simulink model "ModeloMonza"  (R2020b)
settings: Solver=FixedStepAuto  StartTime=0.0  StopTime=7  FixedStep=0.001  RelTol=1e-3
undefined symbols (not defined in the file or in its folder): magnitude
libraries: simulink x2, simulink_extras x1
settings Model: PauseTimes=2.78  Creator=alvar  LastModifiedBy=alvar
settings SolverCC: AlgebraicLoopSolver=LineSearch

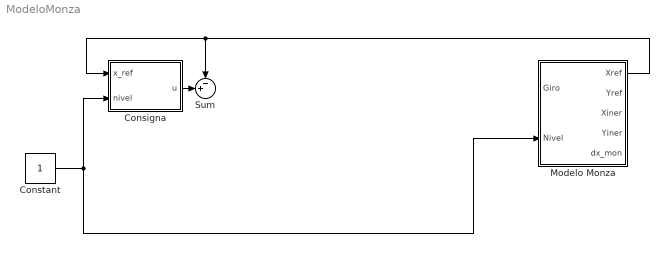
== system ModeloMonza ==
  Consigna : MATLAB Function  TreatAsAtomicUnit=on
  Constant : Constant
  Modelo Monza : Subsystem
  Sum : Sum  Inputs=-+|
  wires:
  Constant/1 -> Modelo Monza/2(Nivel), Consigna/2(nivel)
  Modelo Monza/1(Xref) -> Consigna/1(x_ref), Sum/1
  Consigna/1(u) -> Sum/2

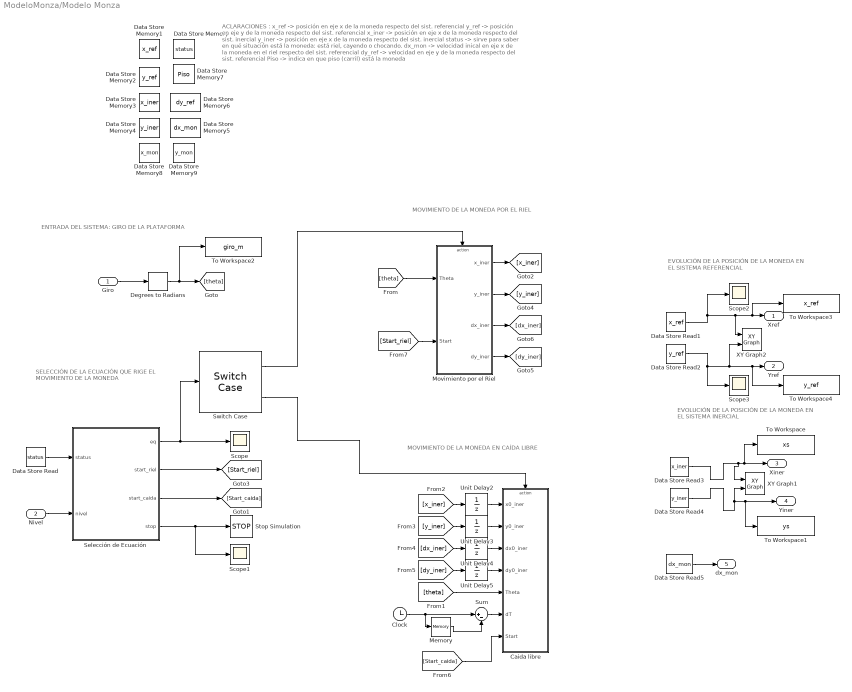
== system ModeloMonza/Modelo Monza ==
  note: ENTRADA DEL SISTEMA: GIRO DE LA PLATAFORMA
  note: SELECCIÓN DE LA ECUACIÓN QUE RIGE EL MOVIMIENTO DE LA MONEDA
  note: MOVIMIENTO DE LA MONEDA EN CAÍDA LIBRE
  note: MOVIMIENTO DE LA MONEDA POR EL RIEL
  note: EVOLUCIÓN DE LA POSICIÓN DE LA MONEDA EN EL SISTEMA REFERENCIAL
  note: ACLARACIONES :
      |
      | x_ref -> posición en eje x de la moneda respecto del sist. referencial
      | y_ref -> posición en eje y de la moneda respecto del sist. referencial
      |
      | x_iner -> posición en eje x de la moneda respecto del sist. inercial
      | y_iner -> posición en eje x de la moneda respecto del sist. inercial
      |
      | status -> sirve para saber en qué situación está la moneda: está riel, cayendo o chocando.
      |
      | dx_mon -> velocidad inical en eje x de la moneda en el riel respecto del sist. referencial
      |
      | dy_ref -> velocidad en eje y de la moneda respecto del sist. referencial
      |
      | Piso -> indica en que piso (carril) está la moneda
  note: EVOLUCIÓN DE LA POSICIÓN DE LA MONEDA EN EL SISTEMA INERCIAL
  Giro : Inport
  Nivel : Inport  Port=2
  Caida libre : Subsystem  TreatAsAtomicUnit=on
  Clock : Clock
  Data Store Memory : DataStoreMemory  DataStoreName=status  ReadBeforeWriteMsg=warning  WriteAfterWriteMsg=warning  WriteAfterReadMsg=warning  ShowAdditionalParam=off  OutDataTypeStr=double
  Data Store Memory1 : DataStoreMemory  DataStoreName=x_ref  ReadBeforeWriteMsg=warning  WriteAfterWriteMsg=warning  WriteAfterReadMsg=warning  InitialValue=-0.11  ShowAdditionalParam=off  OutDataTypeStr=double
  Data Store Memory2 : DataStoreMemory  DataStoreName=y_ref  ReadBeforeWriteMsg=warning  WriteAfterWriteMsg=warning  WriteAfterReadMsg=warning  InitialValue=0.107766  ShowAdditionalParam=off  OutDataTypeStr=double
  Data Store Memory3 : DataStoreMemory  DataStoreName=x_iner  ReadBeforeWriteMsg=warning  WriteAfterWriteMsg=warning  WriteAfterReadMsg=warning  InitialValue=-0.11  ShowAdditionalParam=off  OutDataTypeStr=double
  Data Store Memory4 : DataStoreMemory  DataStoreName=y_iner  ReadBeforeWriteMsg=warning  WriteAfterWriteMsg=warning  WriteAfterReadMsg=warning  InitialValue=0.107766  ShowAdditionalParam=off  OutDataTypeStr=double
  Data Store Memory5 : DataStoreMemory  DataStoreName=dx_mon  ReadBeforeWriteMsg=warning  WriteAfterWriteMsg=warning  WriteAfterReadMsg=warning  ShowAdditionalParam=off  OutDataTypeStr=double
  Data Store Memory6 : DataStoreMemory  DataStoreName=dy_ref  ReadBeforeWriteMsg=warning  WriteAfterWriteMsg=warning  WriteAfterReadMsg=warning  ShowAdditionalParam=off  OutDataTypeStr=double
  Data Store Memory7 : DataStoreMemory  DataStoreName=Piso  ReadBeforeWriteMsg=warning  WriteAfterWriteMsg=warning  WriteAfterReadMsg=warning  InitialValue=1  ShowAdditionalParam=off  OutDataTypeStr=double
  Data Store Memory8 : DataStoreMemory  DataStoreName=x_mon  ReadBeforeWriteMsg=warning  WriteAfterWriteMsg=warning  WriteAfterReadMsg=warning  InitialValue=-0.11  ShowAdditionalParam=off  OutDataTypeStr=double
  Data Store Memory9 : DataStoreMemory  DataStoreName=y_mon  ReadBeforeWriteMsg=warning  WriteAfterWriteMsg=warning  WriteAfterReadMsg=warning  InitialValue=0.107766  ShowAdditionalParam=off  OutDataTypeStr=double
  Data Store Read : DataStoreRead  DataStoreName=status
  Data Store Read1 : DataStoreRead  DataStoreName=x_ref
  Data Store Read2 : DataStoreRead  DataStoreName=y_ref
  Data Store Read3 : DataStoreRead  DataStoreName=x_iner
  Data Store Read4 : DataStoreRead  DataStoreName=y_iner
  Data Store Read5 : DataStoreRead  DataStoreName=dx_mon
  Degrees to Radians : simulink_extras/Transformations/Degrees to Radians
  Memory : Memory
  Movimiento por el Riel : Subsystem  TreatAsAtomicUnit=on
  Scope{,1..3} (4 alike) : Scope
  Selección de Ecuación : MATLAB Function  TreatAsAtomicUnit=on
  Stop Simulation : Stop
  Sum : Sum  Inputs=|+-
  Switch Case : SwitchCase  CaseConditions={1,2}  ShowDefaultCase=off
  To Workspace : ToWorkspace  VariableName=xs  SampleTime=0.01
  To Workspace1 : ToWorkspace  VariableName=ys  SampleTime=0.01
  To Workspace2 : ToWorkspace  VariableName=giro_m  SampleTime=0.01
  To Workspace3 : ToWorkspace  VariableName=x_ref  SampleTime=0.01
  To Workspace4 : ToWorkspace  VariableName=y_ref  SampleTime=0.01
  Unit Delay{2..5} (4 alike) : UnitDelay  SampleTime=-1  HasFrameUpgradeWarning=on
  XY Graph1 : simulink/Sinks/XY Graph  xmin=-0.5  xmax=0.5  ymin=-0.5  ymax=0.5  st=-1
  XY Graph2 : simulink/Sinks/XY Graph  xmin=-0.5  xmax=0.5  ymin=-0.5  ymax=0.5  st=-1
  Xref : Outport
  Yref : Outport  Port=2
  Xiner : Outport  Port=3
  Yiner : Outport  Port=4
  dx_mon : Outport  Port=5
  wires:
  Degrees to Radians/1 -> To Workspace2/1, [theta]
  Unit Delay2/1 -> Caida libre/1(x0_iner)
  Data Store Read3/1 -> XY Graph1/1, To Workspace/1, Xiner/1
  Unit Delay3/1 -> Caida libre/2(y0_iner)
  [x_iner] -> Unit Delay2/1
  Switch Case/1 -> Movimiento por el Riel/Action
  [dx_iner] -> Unit Delay4/1
  [dy_iner] -> Unit Delay5/1
  Switch Case/2 -> Caida libre/Action
  Sum/1 -> Caida libre/6(dT)
  Memory/1 -> Sum/2
  Data Store Read2/1 -> XY Graph2/2, To Workspace4/1, Yref/1, Scope3/1
  [theta] -> Movimiento por el Riel/1(Theta)
  Data Store Read4/1 -> XY Graph1/2, To Workspace1/1, Yiner/1
  [y_iner] -> Unit Delay3/1
  Selección de Ecuación/1(eq) -> Scope/1, Switch Case/1
  Unit Delay5/1 -> Caida libre/4(dy0_iner)
  Selección de Ecuación/3(start_caida) -> [Start_caida]
  Clock/1 -> Sum/1, Memory/1
  Data Store Read1/1 -> Scope2/1, XY Graph2/1, To Workspace3/1, Xref/1
  Movimiento por el Riel/2(y_iner) -> [y_iner]
  Movimiento por el Riel/4(dy_iner) -> [dy_iner]
  Movimiento por el Riel/1(x_iner) -> [x_iner]
  Movimiento por el Riel/3(dx_iner) -> [dx_iner]
  [Start_caida] -> Caida libre/7(Start)
  Nivel/1 -> Selección de Ecuación/2(nivel)
  Data Store Read/1 -> Selección de Ecuación/1(status)
  Selección de Ecuación/2(start_riel) -> [Start_riel]
  [theta] -> Caida libre/5(Theta)
  Selección de Ecuación/4(stop) -> Scope1/1, Stop Simulation/1
  [Start_riel] -> Movimiento por el Riel/2(Start)
  Unit Delay4/1 -> Caida libre/3(dx0_iner)
  Giro/1 -> Degrees to Radians/1
  Data Store Read5/1 -> dx_mon/1

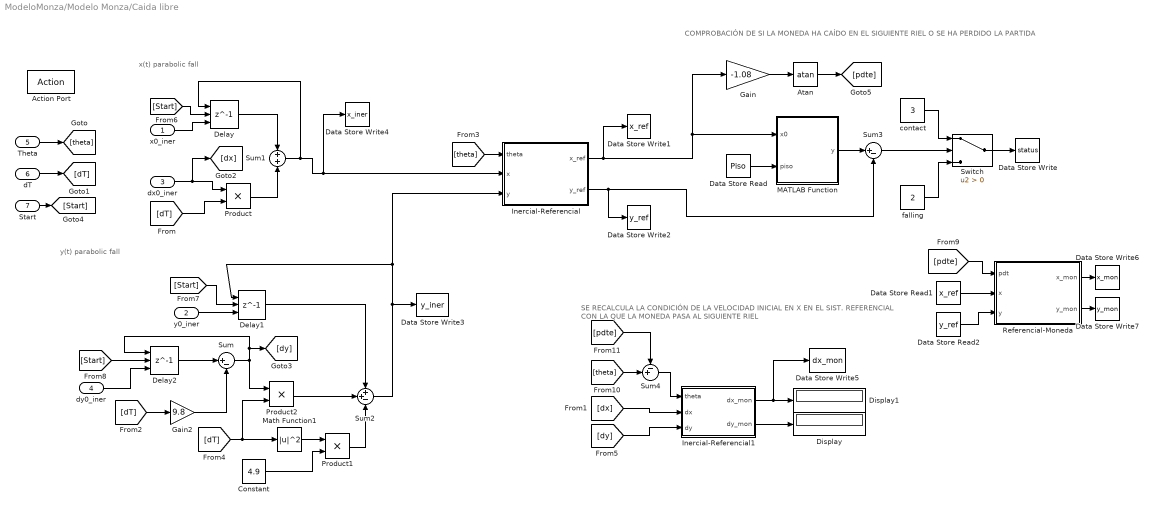
== system ModeloMonza/Modelo Monza/Caida libre ==
  note: SE RECALCULA LA CONDICIÓN DE LA VELOCIDAD INICIAL EN X EN EL SIST. REFERENCIAL CON LA QUE LA MONEDA PASA AL SIGUIENTE RIEL
  note: COMPROBACIÓN DE SI LA MONEDA HA CAÍDO EN EL SIGUIENTE RIEL O SE HA PERDIDO LA PARTIDA
  note: x(t) parabolic fall
  note: y(t) parabolic fall
  x0_iner : Inport
  y0_iner : Inport  Port=2
  dx0_iner : Inport  Port=3
  dy0_iner : Inport  Port=4
  Theta : Inport  Port=5
  dT : Inport  Port=6
  Start : Inport  Port=7
  Action Port : ActionPort  ActionPortLabel=case [ 2 ]:
  Atan : Trigonometry  Operator=atan
  Constant : Constant  Value=4.9
  Data Store Read : DataStoreRead  DataStoreName=Piso
  Data Store Read1 : DataStoreRead  DataStoreName=x_ref
  Data Store Read2 : DataStoreRead  DataStoreName=y_ref
  Data Store Write : DataStoreWrite  DataStoreName=status
  Data Store Write1 : DataStoreWrite  DataStoreName=x_ref
  Data Store Write2 : DataStoreWrite  DataStoreName=y_ref
  Data Store Write3 : DataStoreWrite  DataStoreName=y_iner
  Data Store Write4 : DataStoreWrite  DataStoreName=x_iner
  Data Store Write5 : DataStoreWrite  DataStoreName=dx_mon
  Data Store Write6 : DataStoreWrite  DataStoreName=x_mon
  Data Store Write7 : DataStoreWrite  DataStoreName=y_mon
  Delay : Delay  DelayLength=1  InitialConditionSource=Input port  ExternalReset=Rising
      settings: InputPortMap=u0,r5,p4
  Delay1 : Delay  DelayLength=1  InitialConditionSource=Input port  ExternalReset=Rising
      settings: InputPortMap=u0,r5,p4
  Delay2 : Delay  DelayLength=1  InitialConditionSource=Input port  ExternalReset=Rising
      settings: InputPortMap=u0,r5,p4
  Display : Display
  Display1 : Display
  Gain : Gain  Gain=-1.08
  Gain2 : Gain  Gain=9.8
  Inercial-Referencial : MATLAB Function  TreatAsAtomicUnit=on
  Inercial-Referencial1 : MATLAB Function  TreatAsAtomicUnit=on
  MATLAB Function : MATLAB Function  TreatAsAtomicUnit=on
  Math Function1 : Math  Operator=magnitude^2  SaturateOnIntegerOverflow=on
  Product : Product
  Product1 : Product
  Product2 : Product
  Referencial-Moneda : MATLAB Function  TreatAsAtomicUnit=on
  Sum : Sum  Inputs=|+-
  Sum1 : Sum
  Sum2 : Sum  Inputs=++-
  Sum3 : Sum  Inputs=|+-
  Sum4 : Sum  Inputs=-+|
  Switch : Switch  Criteria=u2 > Threshold
  contact : Constant  Value=3
  falling : Constant  Value=2
  wires:
  [dT] -> Product/2
  Product/1 -> Sum1/2
  Delay1/1 -> Sum2/1
  [dT] -> Product2/2, Math Function1/1
  Sum1/1 -> Data Store Write4/1, Inercial-Referencial/2(x), Delay/1
  Product2/1 -> Sum2/2
  Product1/1 -> Sum2/3
  Math Function1/1 -> Product1/1
  Theta/1 -> [theta]
  x0_iner/1 -> Delay/3
  Delay/1 -> Sum1/1
  dT/1 -> [dT]
  dx0_iner/1 -> Product/1, [dx]
  y0_iner/1 -> Delay1/3
  Sum2/1 -> Inercial-Referencial/3(y), Delay1/1, Data Store Write3/1
  dy0_iner/1 -> Delay2/3
  Delay2/1 -> Sum/1
  [dT] -> Gain2/1
  Gain2/1 -> Sum/2
  Sum/1 -> Product2/1, [dy], Delay2/1
  [theta] -> Inercial-Referencial/1(theta)
  Constant/1 -> Product1/2
  [dx] -> Inercial-Referencial1/2(dx)
  [dy] -> Inercial-Referencial1/3(dy)
  Inercial-Referencial/1(x_ref) -> Gain/1, MATLAB Function/1(x0), Data Store Write1/1
  Data Store Read/1 -> MATLAB Function/2(piso)
  MATLAB Function/1(y) -> Sum3/1
  Inercial-Referencial/2(y_ref) -> Sum3/2, Data Store Write2/1
  falling/1 -> Switch/3
  Sum3/1 -> Switch/2
  Switch/1 -> Data Store Write/1
  contact/1 -> Switch/1
  Inercial-Referencial1/1(dx_mon) -> Data Store Write5/1, Display1/1
  Inercial-Referencial1/2(dy_mon) -> Display/1
  Start/1 -> [Start]
  [Start] -> Delay/2
  [Start] -> Delay1/2
  [Start] -> Delay2/2
  Gain/1 -> Atan/1
  [theta] -> Sum4/2
  [pdte] -> Sum4/1
  Sum4/1 -> Inercial-Referencial1/1(theta)
  Atan/1 -> [pdte]
  [pdte] -> Referencial-Moneda/1(pdt)
  Data Store Read1/1 -> Referencial-Moneda/2(x)
  Data Store Read2/1 -> Referencial-Moneda/3(y)
  Referencial-Moneda/1(x_mon) -> Data Store Write6/1
  Referencial-Moneda/2(y_mon) -> Data Store Write7/1

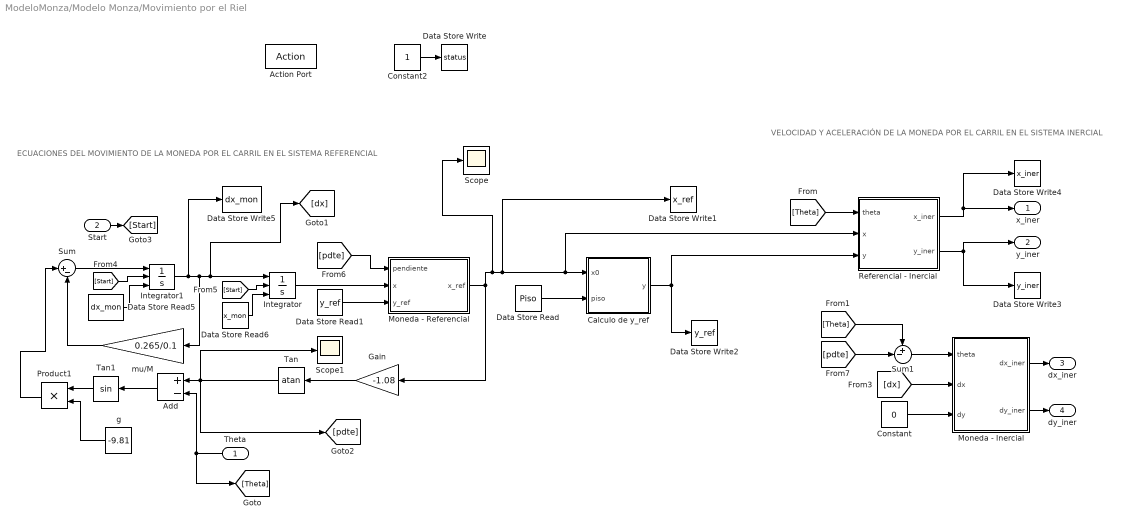
== system ModeloMonza/Modelo Monza/Movimiento por el Riel ==
  note: VELOCIDAD Y ACELERACIÓN DE LA MONEDA POR EL CARRIL EN EL SISTEMA INERCIAL
  note: ECUACIONES DEL MOVIMIENTO DE LA MONEDA POR EL CARRIL EN EL SISTEMA REFERENCIAL
  Theta : Inport
  Start : Inport  Port=2
  Action Port : ActionPort  ActionPortLabel=case [ 1 ]:
  Add : Sum  Inputs=+-
  Calculo de y_ref : MATLAB Function  TreatAsAtomicUnit=on
  Constant : Constant  Value=0
  Constant2 : Constant
  Data Store Read : DataStoreRead  DataStoreName=Piso
  Data Store Read1 : DataStoreRead  DataStoreName=y_ref
  Data Store Read5 : DataStoreRead  DataStoreName=dx_mon
  Data Store Read6 : DataStoreRead  DataStoreName=x_mon
  Data Store Write : DataStoreWrite  DataStoreName=status
  Data Store Write1 : DataStoreWrite  DataStoreName=x_ref
  Data Store Write2 : DataStoreWrite  DataStoreName=y_ref
  Data Store Write3 : DataStoreWrite  DataStoreName=y_iner
  Data Store Write4 : DataStoreWrite  DataStoreName=x_iner
  Data Store Write5 : DataStoreWrite  DataStoreName=dx_mon
  Gain : Gain  Gain=-1.08
  Integrator : Integrator  ExternalReset=rising  InitialConditionSource=external
  Integrator1 : Integrator  ExternalReset=rising  InitialConditionSource=external
  Moneda - Inercial : MATLAB Function  TreatAsAtomicUnit=on
  Moneda - Referencial : MATLAB Function  TreatAsAtomicUnit=on
  Product1 : Product
  Referencial - Inercial : MATLAB Function  TreatAsAtomicUnit=on
  Scope : Scope
  Scope1 : Scope
  Sum : Sum  Inputs=|+-
  Sum1 : Sum  Inputs=+-|
  Tan : Trigonometry  Operator=atan
  Tan1 : Trigonometry
  g : Constant  Value=-9.81
  mu/M : Gain  Gain=0.265/0.1
  x_iner : Outport
  y_iner : Outport  Port=2
  dx_iner : Outport  Port=3
  dy_iner : Outport  Port=4
  wires:
  Add/1 -> Tan1/1
  Tan/1 -> Add/1, Scope1/1, [pdte]
  Gain/1 -> Tan/1
  mu/M/1 -> Sum/2
  g/1 -> Product1/2
  Integrator1/1 -> Data Store Write5/1, mu/M/1, [dx], Integrator/1
  Data Store Read5/1 -> Integrator1/3
  Sum/1 -> Integrator1/1
  Tan1/1 -> Product1/1
  Data Store Read6/1 -> Integrator/3
  Theta/1 -> [Theta], Add/2
  Data Store Read/1 -> Calculo de y_ref/2(piso)
  Calculo de y_ref/1(y) -> Referencial - Inercial/3(y), Data Store Write2/1
  Constant2/1 -> Data Store Write/1
  Referencial - Inercial/1(x_iner) -> Data Store Write4/1, x_iner/1
  Referencial - Inercial/2(y_iner) -> Data Store Write3/1, y_iner/1
  [Theta] -> Referencial - Inercial/1(theta)
  Moneda - Inercial/2(dy_iner) -> dy_iner/1
  Moneda - Inercial/1(dx_iner) -> dx_iner/1
  [dx] -> Moneda - Inercial/2(dx)
  Constant/1 -> Moneda - Inercial/3(dy)
  Start/1 -> [Start]
  [Start] -> Integrator1/2
  [Start] -> Integrator/2
  Integrator/1 -> Moneda - Referencial/2(x)
  Moneda - Referencial/1(x_ref) -> Calculo de y_ref/1(x0), Referencial - Inercial/2(x), Data Store Write1/1, Scope/1, Gain/1
  [pdte] -> Moneda - Referencial/1(pendiente)
  Product1/1 -> Sum/1
  Data Store Read1/1 -> Moneda - Referencial/3(y_ref)
  [Theta] -> Sum1/1
  [pdte] -> Sum1/2
  Sum1/1 -> Moneda - Inercial/1(theta)

== matlab function ModeloMonza/Modelo Monza/Caida libre/Referencial-Moneda ==
  settings: updateMethod=DISCRETE
  data: pdt input; x_mon output; x input; y input; y_mon output
function [x_mon,y_mon] = rotate(pdt,x,y)
x_mon = x*cos(-pdt) + y*sin(-pdt);
y_mon = -x*sin(-pdt) + y*cos(-pdt);

== matlab function ModeloMonza/Modelo Monza/Movimiento por el Riel/Moneda - Referencial ==
  settings: updateMethod=DISCRETE
  data: pendiente input; x_ref output; x input; y_ref input
function x_ref  = rotate(pendiente,x,y_ref)
x_ref_ant = pendiente/-1.08;
y_mon = x_ref_ant*sin(-pendiente)+y_ref*cos(-pendiente);
x_ref =  x*cos(pendiente) + y_mon*sin(pendiente);

== matlab function ModeloMonza/Modelo Monza/Movimiento por el Riel/Calculo de y_ref ==
  data: x0 input; y output; piso input
function y  = fcn(x0, piso)

switch piso
    case 1
        y= -0.54*x0^2 + 0.1143;
    case 2
        y= -0.54*x0^2 + 0.0686;
    case 3
        y= -0.54*x0^2 + 0.03;
    case 4
        y= -0.54*x0^2 - 0.03;  
    case 5
        y= -0.54*x0^2 - 0.0686; 
    case 6
        y= -0.54*x0^2 - 0.1143;
    case 7
        y= -0.54*x0^2 - 0.16;
    otherwise
        y = 0;
end

== matlab function ModeloMonza/Modelo Monza/Caida libre/Inercial-Referencial ==
  settings: updateMethod=DISCRETE
  data: theta input; x_ref output; x input; y input; y_ref output
function [x_ref,y_ref] = rotate(theta,x,y)
x_ref = x*cos(theta) - y*sin(theta);
y_ref = x*sin(theta) + y*cos(theta);

== matlab function ModeloMonza/Modelo Monza/Selección de Ecuación ==
  settings: updateMethod=DISCRETE
  data: eq output; status input; x_ref data_store_memory; Piso data_store_memory; start_riel output; start_caida output; stop output; nivel input
function [eq, start_riel, start_caida, stop] = fcn(status, nivel)

%%DE MOMENTO ESTE CÓDIGO ES PARA PROBAR LAS ECUACIONES EN LA PRIMERA CAIDA
persistent x_edges
persistent equation
global x_ref;
global Piso;
start_riel = 0;
start_caida = 0;
stop = 0;
if(isempty(equation))
    equation = 1;
end
coder.extrinsic('fallCoor');
if (isempty(x_edges))
    x_edges = zeros(7,2);
    x_edges = fallCoor(nivel);
end
%x_edges = fallCoor(1)

if(status == 1)
    switch Piso
        case 1
            if (x_ref > x_edges(1,1)) % empieza a caer
              equation = 2; % se utiliza las ecuaciones de caída libre
              start_caida = 1; % se resetean los bloques delay
            elseif (x_ref < x_edges(1,2))
                stop = 1;
            end
        case 2
            if (x_ref < x_edges(2,2))
                equation = 2;
                start_caida = 1;
            elseif (x_ref > x_edges(2,1))
                stop = 1;
            end
        case 3
            if (x_ref > x_edges(3,1))
                equation = 2;
                start_caida = 1;
            elseif (x_ref < x_edges(3,2))
                stop = 1;
            end
        case 4
            if (x_ref < x_edges(4,2))
                equation = 2;
                start_caida = 1;
            elseif (x_ref > x_edges(4,1))
                stop = 1;
            end
        case 5
            if (x_ref > x_edges(5,1))
                equation = 2;
                start_caida = 1;
            elseif (x_ref < x_edges(5,2))
                stop = 1;
            end
        case 6
            if (x_ref < x_edges(6,2))
                equation = 2;
                start_caida = 1;
            elseif (x_ref > x_edges(6,1))
                stop = 1;
            end
        case 7
            if (x_ref > x_edges(7,1))
                equation = 2;
                start_caida = 1;
            elseif (x_ref < x_edges(7,2))
                stop = 1;
            end
    end
end


if(status == 2)
    switch Piso   
        case 1
            if (x_ref > x_edges(2,1))
                stop = 1;
            end
        case 2
            if (x_ref < x_edges(3,2))
                stop = 1;
            end
        case 3
            if (x_ref > x_edges(4,1))
                stop = 1;
            end
        case 4
            if (x_ref < x_edges(5,2))
                stop = 1;
            end
        case 5
            if (x_ref > x_edges(6,1))
                stop = 1;
            end
        case 6
            if (x_ref > x_edges(7,1))
                stop = 1;
            elseif (x_ref < x_edges(7,2))
                stop = 1;
            end 
    end   
end



if(status == 3) % impacto
    equation = 1; % se utiliza el bloque movimiento por el riel
    Piso = Piso + 1; % se pasa al siguiente piso
    start_riel = 1; % se reseta el integrador 
end

eq = equation;

== matlab function ModeloMonza/Modelo Monza/Caida libre/Inercial-Referencial1 ==
  settings: updateMethod=DISCRETE
  data: theta input; dx_mon output; dx input; dy input; dy_mon output
function [dx_mon,dy_mon] = rotate(theta,dx,dy)
dx_mon = dx*cos(theta) + dy*sin(theta);
dy_mon = -dx*sin(theta) + dy*cos(theta);

== matlab function ModeloMonza/Consigna ==
  settings: updateMethod=DISCRETE
  data: x_ref input; nivel input; u output
function u = fcn(x_ref, nivel)

persistent piso 
persistent x_edge

if isempty(piso)
    piso = 1;
end

coder.extrinsic('fallCoor');
if (isempty(x_edge))
    x_edge = zeros(7,2);
    x_edge = fallCoor(nivel);
end

switch piso
    case 1
        u = x_edge(1,1)+0.01;
        if(x_ref > x_edge(1,1))
            piso = piso + 1;
        end
    case 2
        u = x_edge(2,2)-0.01;
        if(x_ref < x_edge(2,2))
            piso = piso + 1;
        end
    case 3
        u = x_edge(3,1)+0.01;
        if(x_ref > x_edge(3,1))
            piso = piso + 1;
        end
    case 4
        u = x_edge(4,2)-0.01;
        if(x_ref < x_edge(4,2))
            piso = piso + 1;
        end 
    case 5
        u = x_edge(5,1)+0.01;
        if(x_ref > x_edge(5,1))
            piso = piso + 1;
        end 
    case 6
        u = x_edge(6,2)-0.01;
        if(x_ref < x_edge(6,2))
            piso = piso + 1;
        end 
    case 7
        u = x_edge(7,1)+0.01;
        if(x_ref > x_edge(7,1))
            piso = piso + 1;
        end
    otherwise
        u = 0;
end

== matlab function ModeloMonza/Modelo Monza/Caida libre/MATLAB Function ==
  data: x0 input; y output; piso input
function y  = fcn(x0, piso)

paux = piso+1;
switch paux
    case 1
        y= -0.54*x0^2 + 0.1143;
    case 2
        y= -0.54*x0^2 + 0.0686;
    case 3
        y= -0.54*x0^2 + 0.03;
    case 4
        y= -0.54*x0^2 - 0.03;
    case 5
        y= -0.54*x0^2 - 0.0686; 
    case 6
        y= -0.54*x0^2 - 0.1143;
    case 7
        y= -0.54*x0^2 - 0.16;
    otherwise
        y = 0;
end

== matlab function ModeloMonza/Modelo Monza/Movimiento por el Riel/Referencial - Inercial ==
  settings: updateMethod=DISCRETE
  data: theta input; x_iner output; x input; y input; y_iner output
function [x_iner,y_iner] = rotate(theta,x,y)
x_iner =  x*cos(theta) + y*sin(theta);
y_iner = -x*sin(theta) + y*cos(theta);

== matlab function ModeloMonza/Modelo Monza/Movimiento por el Riel/Moneda - Inercial ==
  settings: updateMethod=DISCRETE
  data: theta input; dx_iner output; dx input; dy input; dy_iner output
function [dx_iner,dy_iner] = rotate(theta,dx,dy)
dx_iner =  dx*cos(theta) + dy*sin(theta);
dy_iner = -dx*sin(theta) + dy*cos(theta);
